simulink model "Ac_DC_two"  (R2017b)
settings: Solver=VariableStepAuto  StartTime=0.0  StopTime=0.1  MaxStep=1e-4  RelTol=1e-3
libraries: powerlib x10, powerlib_meascontrol x1
settings Model: Creator=DELL  LastModifiedBy=DELL

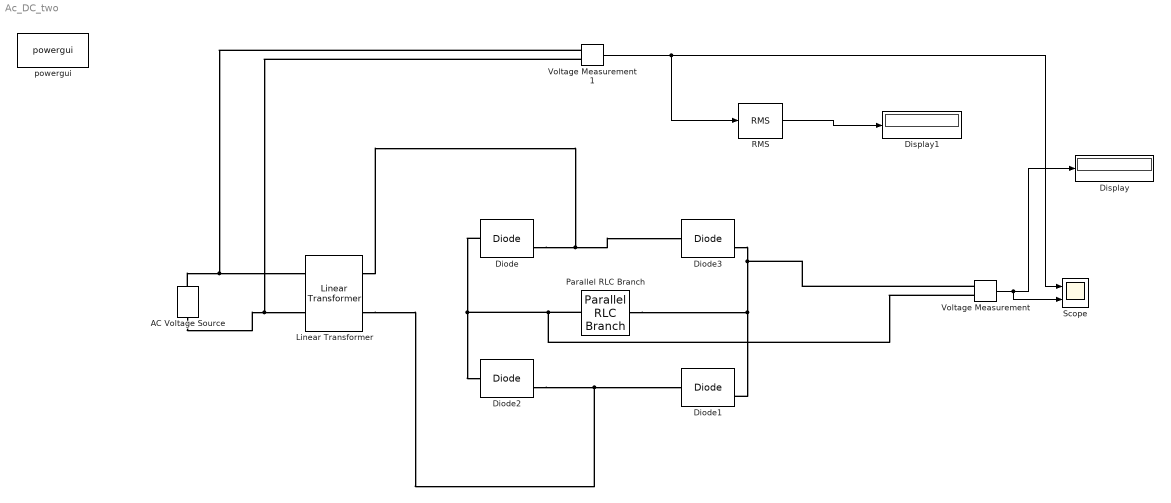
== system Ac_DC_two ==
  AC Voltage Source : powerlib/Electrical Sources/AC Voltage Source  Amplitude=230  Phase=0  Frequency=50  SampleTime=0  Measurements=None  BusType=swing  Pref=10e3  Qref=0  Qmin=-inf  Qmax=+inf
  Diode{,1..3} (4 alike) : powerlib/Power Electronics/Diode  Ron=0.001  Lon=0  Vf=0  IC=0  UseSnubber=0  Rs=inf  Cs=inf  Measurements=on
  Display : Display
  Display1 : Display
  Linear Transformer : powerlib/Elements/Linear Transformer  UNITS=pu  NominalPower=[ 250e6 50 ]  winding1="[ 230  0  0 ]"  winding2="[ 12  0  0 ]"  ThreeWindings=off  winding3=[ 315e3 0.002 0.08 ]  RmLm=[ 500 500 ]  Measurements=None  DataType=off
  Parallel RLC Branch : powerlib/Elements/Parallel RLC Branch  LConnTagsString=a  RConnTagsString=__new0  BranchType=RC  Resistance=1000  Inductance=1e-3  SetiL0=off  InitialCurrent=0  Capacitance=1e-2  Setx0=off  InitialVoltage=0  Measurements=None
  RMS : powerlib_meascontrol/Measurements/RMS  TrueRMS=on  Freq=50  RMSInit=0  Ts=0
  Scope : Scope  NumInputPorts=2
  Voltage Measurement : powerlib/Measurements/Voltage Measurement  PhasorSimulation=off  OutputType=Complex  PSBequivalent=0
  Voltage Measurement1 : powerlib/Measurements/Voltage Measurement  PhasorSimulation=off  OutputType=Complex  PSBequivalent=0
  powergui : powerlib/powergui  Priority=1  SimulationMode=Continuous  SampleTime=50e-6  frequency=60  Iterations=50  frequencyindice=50  Pbase=100e6  ErrMax=1e-4  UnitsV=kV  UnitsW=MW  buscounter=0  FunctionMessages=off  echomessages=off  EnableUseOfTLC=off  CurrentSourceSwitches=off  DisableSnubberDevices=off  DisableRonSwitches=off  DisableVfSwitches=off  DisplayEquations=off  SolverType=Tustin/Backward Euler (TBE)  Interpol=off  ExternalGateDelay=off  methode=off  Ts=100  x0status=blocks  SPID=on  SwTol=0  HookPort=off  RestoreLinks=warning  ResistiveCurrentMeasurement=off  Frange=[0:2:500]  Ylog=off  Xlog=on  ShowGrid=off  save=off  variable=ZData  structure=0  ZoomFFT=off  StartTime=0.0  cycles=1  DisplayStyle=1  fundamental=60  FreqAxis=off  MaxFrequency=1000  frequencyindicesteady=1  RmsSteady=1  display=off
  wires:
  Voltage Measurement/1 -> Scope/2, Display/1
  Voltage Measurement1/1 -> RMS/1, Scope/1
  RMS/1 -> Display1/1
  connections:
  Diode/RConn1 -- Linear Transformer/RConn1 -- Diode3/LConn1
  Diode3/RConn1 -- Voltage Measurement/LConn1 -- Parallel RLC Branch/RConn1 -- Diode1/RConn1
  Diode2/RConn1 -- Linear Transformer/RConn2 -- Diode1/LConn1
  Diode/LConn1 -- Voltage Measurement/LConn2 -- Parallel RLC Branch/LConn1 -- Diode2/LConn1
  AC Voltage Source/RConn1 -- Voltage Measurement1/LConn1 -- Linear Transformer/LConn1
  AC Voltage Source/LConn1 -- Voltage Measurement1/LConn2 -- Linear Transformer/LConn2
